simulink model "BEST2020_Autonomous_7thGraders"  (R2021a)
settings: Solver=ode23t  StartTime=0.0  StopTime=120.1  FixedStep=0.05  RelTol=1e-3  EnableMultiTasking=on
model workspace (MAT data in the model file):
  mapForSim : object (value not decoded)
  occGrid : robotics.BinaryOccupancyGrid (value not decoded)
values from neighbouring files (symbols this model uses):
  cellLevel = [0 0 0 1 0 0 0 0 0 0 0 0 0 0 0 0 0 0 1 0 0 ]    [BEST2020GameConfigAuto1.m]    (also in BEST2020GameConfigAuto2.m; BEST2020GameConfigAuto3.m)
  cellPose = [0.920 1.265;     1.035 1.380;     0.805 1.380;     0.920 0.920;     1.035 0.920;     0.805 0.920;     1.035 0.460;     0.920 0.575;     0.805 0.575;     0.575 0.000;     0.460 0.115;     0.345 0.000;     0.805 -0.460;     1.035 -0.460;     0.920 -0.460;     0.920 -0.805;     0.805 -0.920;     1.035 -1.035;     1.265 -1.265;     1.380 -1.380;     1.495 -1.265]    [BEST2020GameConfigAuto1.m]    (also in BEST2020GameConfigAuto2.m; BEST2020GameConfigAuto3.m)
  cellTypeArray = [0 0 0 0 0 0 0 0 0 0 0 0 0 0 0 0 0 0 0 0 0 ]    [BEST2020GameConfigAuto1.m]    (also in BEST2020GameConfigAuto2.m = [1 1 1 1 2 1 2 2 2 2 1 2 1 2 2 1 1 1 1 2 2 ]; BEST2020GameConfigAuto3.m = [0 0 1 1 0 0 0 1 2 0 0 1 0 0 1 0 0 2 2 0 1 ])
  isoPoses = [0.91 0;-0.91/2 0.91;-0.91/2 -0.91]    [BEST2020GameConfigAuto1.m]    (also in BEST2020GameConfigAuto2.m; BEST2020GameConfigAuto3.m)
  platformPoses = [0.91 0.91;1.37 -1.37]    [BEST2020GameConfigAuto1.m]    (also in BEST2020GameConfigAuto2.m; BEST2020GameConfigAuto3.m)
undefined symbols (not defined in the file or in its folder): FloorSurface, PlowSurface, Ref, RobotSurface, WallSurface, X, Y, Z
libraries: sm_lib x286, nesl_utility x157, simulink x72
(part 15 of 15)

== matlab function BEST2020_Autonomous_7thGraders/BEST Robotics 2020 Game (Double-Click)1/Cells/Object18/MATLAB Function ==
  settings: updateMethod=DISCRETE
  data: latch input; scoreLevel input; inuse input; target input; time input; objPoseX output; robotPoseX input; robotPoseY input; objPoseY output; latched output; initPose parameter; objId parameter; cellType output; endType output; cellTypeArray parameter; gameTime parameter; platformPoses parameter; cellLevel parameter
function [objPoseX, objPoseY, latched, cellType,endType] = latchObject(latch,scoreLevel, inuse, target, time, robotPoseX, robotPoseY, initPose, objId, cellTypeArray, gameTime, platformPoses, cellLevel)
persistent stateX stateY level pickup
if isempty(stateX)
    stateX=initPose(1);
    stateY=initPose(2);
    level=cellLevel;
    pickup=0;
end

if ~latch
     pickup=0;
    if level && ((stateX > platformPoses(1,1)-0.21 && stateX < platformPoses(1,1)+0.21...
            && stateY > platformPoses(1,2)-0.21 && stateY < platformPoses(1,2) +0.21) || ...
            (stateX > platformPoses(2,1)-0.21 && stateX < platformPoses(2,1)+0.21...
            && stateY > platformPoses(2,2)-0.21 && stateY < platformPoses(2,2) +0.21))
        latched=0.4;
    else
        level=0;
        latched=0;
    end
elseif pickup
    stateX=robotPoseX;
    stateY=robotPoseY;
    level=scoreLevel;
    latched=0.15 +level*0.4;
elseif ~inuse && latch && target == objId && ...
        sqrt((stateX-robotPoseX)^2+(stateY-robotPoseY)^2) < 0.08 && scoreLevel==level
    
        pickup=1;
        latched=0.15;
else
   if level && ((stateX > platformPoses(1,1)-0.21 && stateX < platformPoses(1,1)+0.21...
            && stateY > platformPoses(1,2)-0.21 && stateY < platformPoses(1,2) +0.21) || ...
            (stateX > platformPoses(2,1)-0.21 && stateX < platformPoses(2,1)+0.21...
            && stateY > platformPoses(2,2)-0.21 && stateY < platformPoses(2,2) +0.21))
        latched=0.4;
    else
        level=0;
        latched=0;
    end
end
if sqrt((stateX-robotPoseX)^2+(stateY-robotPoseY)^2) < 0.1 && scoreLevel==level
    cellType=cellTypeArray(objId);
else
    cellType=nan;
end

if time > gameTime
    endType=cellTypeArray(objId)+1;
else
    endType=0;
end

objPoseX=stateX;
objPoseY=stateY;

== matlab function BEST2020_Autonomous_7thGraders/BEST Robotics 2020 Game (Double-Click)1/Cells/Object19/MATLAB Function ==
  settings: updateMethod=DISCRETE
  data: latch input; scoreLevel input; inuse input; target input; time input; objPoseX output; robotPoseX input; robotPoseY input; objPoseY output; latched output; initPose parameter; objId parameter; cellType output; endType output; cellTypeArray parameter; gameTime parameter; platformPoses parameter; cellLevel parameter
function [objPoseX, objPoseY, latched, cellType,endType] = latchObject(latch,scoreLevel, inuse, target, time, robotPoseX, robotPoseY, initPose, objId, cellTypeArray, gameTime, platformPoses, cellLevel)
persistent stateX stateY level pickup
if isempty(stateX)
    stateX=initPose(1);
    stateY=initPose(2);
    level=cellLevel;
    pickup=0;
end

if ~latch
     pickup=0;
    if level && ((stateX > platformPoses(1,1)-0.21 && stateX < platformPoses(1,1)+0.21...
            && stateY > platformPoses(1,2)-0.21 && stateY < platformPoses(1,2) +0.21) || ...
            (stateX > platformPoses(2,1)-0.21 && stateX < platformPoses(2,1)+0.21...
            && stateY > platformPoses(2,2)-0.21 && stateY < platformPoses(2,2) +0.21))
        latched=0.4;
    else
        level=0;
        latched=0;
    end
elseif pickup
    stateX=robotPoseX;
    stateY=robotPoseY;
    level=scoreLevel;
    latched=0.15 +level*0.4;
elseif ~inuse && latch && target == objId && ...
        sqrt((stateX-robotPoseX)^2+(stateY-robotPoseY)^2) < 0.08 && scoreLevel==level
    
        pickup=1;
        latched=0.15;
else
   if level && ((stateX > platformPoses(1,1)-0.21 && stateX < platformPoses(1,1)+0.21...
            && stateY > platformPoses(1,2)-0.21 && stateY < platformPoses(1,2) +0.21) || ...
            (stateX > platformPoses(2,1)-0.21 && stateX < platformPoses(2,1)+0.21...
            && stateY > platformPoses(2,2)-0.21 && stateY < platformPoses(2,2) +0.21))
        latched=0.4;
    else
        level=0;
        latched=0;
    end
end
if sqrt((stateX-robotPoseX)^2+(stateY-robotPoseY)^2) < 0.1 && scoreLevel==level
    cellType=cellTypeArray(objId);
else
    cellType=nan;
end

if time > gameTime
    endType=cellTypeArray(objId)+1;
else
    endType=0;
end

objPoseX=stateX;
objPoseY=stateY;

== matlab function BEST2020_Autonomous_7thGraders/BEST Robotics 2020 Game (Double-Click)1/Cells/Object2/MATLAB Function ==
  settings: updateMethod=DISCRETE
  data: latch input; scoreLevel input; inuse input; target input; time input; objPoseX output; robotPoseX input; robotPoseY input; objPoseY output; latched output; initPose parameter; objId parameter; cellType output; endType output; cellTypeArray parameter; gameTime parameter; platformPoses parameter; cellLevel parameter
function [objPoseX, objPoseY, latched, cellType,endType] = latchObject(latch,scoreLevel, inuse, target, time, robotPoseX, robotPoseY, initPose, objId, cellTypeArray, gameTime, platformPoses, cellLevel)
persistent stateX stateY level pickup
if isempty(stateX)
    stateX=initPose(1);
    stateY=initPose(2);
    level=cellLevel;
    pickup=0;
end

if ~latch
     pickup=0;
    if level && ((stateX > platformPoses(1,1)-0.21 && stateX < platformPoses(1,1)+0.21...
            && stateY > platformPoses(1,2)-0.21 && stateY < platformPoses(1,2) +0.21) || ...
            (stateX > platformPoses(2,1)-0.21 && stateX < platformPoses(2,1)+0.21...
            && stateY > platformPoses(2,2)-0.21 && stateY < platformPoses(2,2) +0.21))
        latched=0.4;
    else
        level=0;
        latched=0;
    end
elseif pickup
    stateX=robotPoseX;
    stateY=robotPoseY;
    level=scoreLevel;
    latched=0.15 +level*0.4;
elseif ~inuse && latch && target == objId && ...
        sqrt((stateX-robotPoseX)^2+(stateY-robotPoseY)^2) < 0.08 && scoreLevel==level
    
        pickup=1;
        latched=0.15;
else
   if level && ((stateX > platformPoses(1,1)-0.21 && stateX < platformPoses(1,1)+0.21...
            && stateY > platformPoses(1,2)-0.21 && stateY < platformPoses(1,2) +0.21) || ...
            (stateX > platformPoses(2,1)-0.21 && stateX < platformPoses(2,1)+0.21...
            && stateY > platformPoses(2,2)-0.21 && stateY < platformPoses(2,2) +0.21))
        latched=0.4;
    else
        level=0;
        latched=0;
    end
end
if sqrt((stateX-robotPoseX)^2+(stateY-robotPoseY)^2) < 0.1 && scoreLevel==level
    cellType=cellTypeArray(objId);
else
    cellType=nan;
end

if time > gameTime
    endType=cellTypeArray(objId)+1;
else
    endType=0;
end

objPoseX=stateX;
objPoseY=stateY;

== matlab function BEST2020_Autonomous_7thGraders/BEST Robotics 2020 Game (Double-Click)1/Cells/Object20/MATLAB Function ==
  settings: updateMethod=DISCRETE
  data: latch input; scoreLevel input; inuse input; target input; time input; objPoseX output; robotPoseX input; robotPoseY input; objPoseY output; latched output; initPose parameter; objId parameter; cellType output; endType output; cellTypeArray parameter; gameTime parameter; platformPoses parameter; cellLevel parameter
function [objPoseX, objPoseY, latched, cellType,endType] = latchObject(latch,scoreLevel, inuse, target, time, robotPoseX, robotPoseY, initPose, objId, cellTypeArray, gameTime, platformPoses, cellLevel)
persistent stateX stateY level pickup
if isempty(stateX)
    stateX=initPose(1);
    stateY=initPose(2);
    level=cellLevel;
    pickup=0;
end

if ~latch
     pickup=0;
    if level && ((stateX > platformPoses(1,1)-0.21 && stateX < platformPoses(1,1)+0.21...
            && stateY > platformPoses(1,2)-0.21 && stateY < platformPoses(1,2) +0.21) || ...
            (stateX > platformPoses(2,1)-0.21 && stateX < platformPoses(2,1)+0.21...
            && stateY > platformPoses(2,2)-0.21 && stateY < platformPoses(2,2) +0.21))
        latched=0.4;
    else
        level=0;
        latched=0;
    end
elseif pickup
    stateX=robotPoseX;
    stateY=robotPoseY;
    level=scoreLevel;
    latched=0.15 +level*0.4;
elseif ~inuse && latch && target == objId && ...
        sqrt((stateX-robotPoseX)^2+(stateY-robotPoseY)^2) < 0.08 && scoreLevel==level
    
        pickup=1;
        latched=0.15;
else
   if level && ((stateX > platformPoses(1,1)-0.21 && stateX < platformPoses(1,1)+0.21...
            && stateY > platformPoses(1,2)-0.21 && stateY < platformPoses(1,2) +0.21) || ...
            (stateX > platformPoses(2,1)-0.21 && stateX < platformPoses(2,1)+0.21...
            && stateY > platformPoses(2,2)-0.21 && stateY < platformPoses(2,2) +0.21))
        latched=0.4;
    else
        level=0;
        latched=0;
    end
end
if sqrt((stateX-robotPoseX)^2+(stateY-robotPoseY)^2) < 0.1 && scoreLevel==level
    cellType=cellTypeArray(objId);
else
    cellType=nan;
end

if time > gameTime
    endType=cellTypeArray(objId)+1;
else
    endType=0;
end

objPoseX=stateX;
objPoseY=stateY;

== matlab function BEST2020_Autonomous_7thGraders/BEST Robotics 2020 Game (Double-Click)1/Cells/Object21/MATLAB Function ==
  settings: updateMethod=DISCRETE
  data: latch input; scoreLevel input; inuse input; target input; time input; objPoseX output; robotPoseX input; robotPoseY input; objPoseY output; latched output; initPose parameter; objId parameter; cellType output; endType output; cellTypeArray parameter; gameTime parameter; platformPoses parameter; cellLevel parameter
function [objPoseX, objPoseY, latched, cellType,endType] = latchObject(latch,scoreLevel, inuse, target, time, robotPoseX, robotPoseY, initPose, objId, cellTypeArray, gameTime, platformPoses, cellLevel)
persistent stateX stateY level pickup
if isempty(stateX)
    stateX=initPose(1);
    stateY=initPose(2);
    level=cellLevel;
    pickup=0;
end

if ~latch
     pickup=0;
    if level && ((stateX > platformPoses(1,1)-0.21 && stateX < platformPoses(1,1)+0.21...
            && stateY > platformPoses(1,2)-0.21 && stateY < platformPoses(1,2) +0.21) || ...
            (stateX > platformPoses(2,1)-0.21 && stateX < platformPoses(2,1)+0.21...
            && stateY > platformPoses(2,2)-0.21 && stateY < platformPoses(2,2) +0.21))
        latched=0.4;
    else
        level=0;
        latched=0;
    end
elseif pickup
    stateX=robotPoseX;
    stateY=robotPoseY;
    level=scoreLevel;
    latched=0.15 +level*0.4;
elseif ~inuse && latch && target == objId && ...
        sqrt((stateX-robotPoseX)^2+(stateY-robotPoseY)^2) < 0.08 && scoreLevel==level
    
        pickup=1;
        latched=0.15;
else
   if level && ((stateX > platformPoses(1,1)-0.21 && stateX < platformPoses(1,1)+0.21...
            && stateY > platformPoses(1,2)-0.21 && stateY < platformPoses(1,2) +0.21) || ...
            (stateX > platformPoses(2,1)-0.21 && stateX < platformPoses(2,1)+0.21...
            && stateY > platformPoses(2,2)-0.21 && stateY < platformPoses(2,2) +0.21))
        latched=0.4;
    else
        level=0;
        latched=0;
    end
end
if sqrt((stateX-robotPoseX)^2+(stateY-robotPoseY)^2) < 0.1 && scoreLevel==level
    cellType=cellTypeArray(objId);
else
    cellType=nan;
end

if time > gameTime
    endType=cellTypeArray(objId)+1;
else
    endType=0;
end

objPoseX=stateX;
objPoseY=stateY;

== matlab function BEST2020_Autonomous_7thGraders/BEST Robotics 2020 Game (Double-Click)1/Cells/Object3/MATLAB Function ==
  settings: updateMethod=DISCRETE
  data: latch input; scoreLevel input; inuse input; target input; time input; objPoseX output; robotPoseX input; robotPoseY input; objPoseY output; latched output; initPose parameter; objId parameter; cellType output; endType output; cellTypeArray parameter; gameTime parameter; platformPoses parameter; cellLevel parameter
function [objPoseX, objPoseY, latched, cellType,endType] = latchObject(latch,scoreLevel, inuse, target, time, robotPoseX, robotPoseY, initPose, objId, cellTypeArray, gameTime, platformPoses, cellLevel)
persistent stateX stateY level pickup
if isempty(stateX)
    stateX=initPose(1);
    stateY=initPose(2);
    level=cellLevel;
    pickup=0;
end

if ~latch
     pickup=0;
    if level && ((stateX > platformPoses(1,1)-0.21 && stateX < platformPoses(1,1)+0.21...
            && stateY > platformPoses(1,2)-0.21 && stateY < platformPoses(1,2) +0.21) || ...
            (stateX > platformPoses(2,1)-0.21 && stateX < platformPoses(2,1)+0.21...
            && stateY > platformPoses(2,2)-0.21 && stateY < platformPoses(2,2) +0.21))
        latched=0.4;
    else
        level=0;
        latched=0;
    end
elseif pickup
    stateX=robotPoseX;
    stateY=robotPoseY;
    level=scoreLevel;
    latched=0.15 +level*0.4;
elseif ~inuse && latch && target == objId && ...
        sqrt((stateX-robotPoseX)^2+(stateY-robotPoseY)^2) < 0.08 && scoreLevel==level
    
        pickup=1;
        latched=0.15;
else
   if level && ((stateX > platformPoses(1,1)-0.21 && stateX < platformPoses(1,1)+0.21...
            && stateY > platformPoses(1,2)-0.21 && stateY < platformPoses(1,2) +0.21) || ...
            (stateX > platformPoses(2,1)-0.21 && stateX < platformPoses(2,1)+0.21...
            && stateY > platformPoses(2,2)-0.21 && stateY < platformPoses(2,2) +0.21))
        latched=0.4;
    else
        level=0;
        latched=0;
    end
end
if sqrt((stateX-robotPoseX)^2+(stateY-robotPoseY)^2) < 0.1 && scoreLevel==level
    cellType=cellTypeArray(objId);
else
    cellType=nan;
end

if time > gameTime
    endType=cellTypeArray(objId)+1;
else
    endType=0;
end

objPoseX=stateX;
objPoseY=stateY;

== matlab function BEST2020_Autonomous_7thGraders/BEST Robotics 2020 Game (Double-Click)1/Cells/Object4/MATLAB Function ==
  settings: updateMethod=DISCRETE
  data: latch input; scoreLevel input; inuse input; target input; time input; objPoseX output; robotPoseX input; robotPoseY input; objPoseY output; latched output; initPose parameter; objId parameter; cellType output; endType output; cellTypeArray parameter; gameTime parameter; platformPoses parameter; cellLevel parameter
function [objPoseX, objPoseY, latched, cellType,endType] = latchObject(latch,scoreLevel, inuse, target, time, robotPoseX, robotPoseY, initPose, objId, cellTypeArray, gameTime, platformPoses, cellLevel)
persistent stateX stateY level pickup
if isempty(stateX)
    stateX=initPose(1);
    stateY=initPose(2);
    level=cellLevel;
    pickup=0;
end

if ~latch
     pickup=0;
    if level && ((stateX > platformPoses(1,1)-0.21 && stateX < platformPoses(1,1)+0.21...
            && stateY > platformPoses(1,2)-0.21 && stateY < platformPoses(1,2) +0.21) || ...
            (stateX > platformPoses(2,1)-0.21 && stateX < platformPoses(2,1)+0.21...
            && stateY > platformPoses(2,2)-0.21 && stateY < platformPoses(2,2) +0.21))
        latched=0.4;
    else
        level=0;
        latched=0;
    end
elseif pickup
    stateX=robotPoseX;
    stateY=robotPoseY;
    level=scoreLevel;
    latched=0.15 +level*0.4;
elseif ~inuse && latch && target == objId && ...
        sqrt((stateX-robotPoseX)^2+(stateY-robotPoseY)^2) < 0.08 && scoreLevel==level
    
        pickup=1;
        latched=0.15;
else
   if level && ((stateX > platformPoses(1,1)-0.21 && stateX < platformPoses(1,1)+0.21...
            && stateY > platformPoses(1,2)-0.21 && stateY < platformPoses(1,2) +0.21) || ...
            (stateX > platformPoses(2,1)-0.21 && stateX < platformPoses(2,1)+0.21...
            && stateY > platformPoses(2,2)-0.21 && stateY < platformPoses(2,2) +0.21))
        latched=0.4;
    else
        level=0;
        latched=0;
    end
end
if sqrt((stateX-robotPoseX)^2+(stateY-robotPoseY)^2) < 0.1 && scoreLevel==level
    cellType=cellTypeArray(objId);
else
    cellType=nan;
end

if time > gameTime
    endType=cellTypeArray(objId)+1;
else
    endType=0;
end

objPoseX=stateX;
objPoseY=stateY;

== matlab function BEST2020_Autonomous_7thGraders/BEST Robotics 2020 Game (Double-Click)1/Cells/Object5/MATLAB Function ==
  settings: updateMethod=DISCRETE
  data: latch input; scoreLevel input; inuse input; target input; time input; objPoseX output; robotPoseX input; robotPoseY input; objPoseY output; latched output; initPose parameter; objId parameter; cellType output; endType output; cellTypeArray parameter; gameTime parameter; platformPoses parameter; cellLevel parameter
function [objPoseX, objPoseY, latched, cellType,endType] = latchObject(latch,scoreLevel, inuse, target, time, robotPoseX, robotPoseY, initPose, objId, cellTypeArray, gameTime, platformPoses, cellLevel)
persistent stateX stateY level pickup
if isempty(stateX)
    stateX=initPose(1);
    stateY=initPose(2);
    level=cellLevel;
    pickup=0;
end

if ~latch
     pickup=0;
    if level && ((stateX > platformPoses(1,1)-0.21 && stateX < platformPoses(1,1)+0.21...
            && stateY > platformPoses(1,2)-0.21 && stateY < platformPoses(1,2) +0.21) || ...
            (stateX > platformPoses(2,1)-0.21 && stateX < platformPoses(2,1)+0.21...
            && stateY > platformPoses(2,2)-0.21 && stateY < platformPoses(2,2) +0.21))
        latched=0.4;
    else
        level=0;
        latched=0;
    end
elseif pickup
    stateX=robotPoseX;
    stateY=robotPoseY;
    level=scoreLevel;
    latched=0.15 +level*0.4;
elseif ~inuse && latch && target == objId && ...
        sqrt((stateX-robotPoseX)^2+(stateY-robotPoseY)^2) < 0.08 && scoreLevel==level
    
        pickup=1;
        latched=0.15;
else
   if level && ((stateX > platformPoses(1,1)-0.21 && stateX < platformPoses(1,1)+0.21...
            && stateY > platformPoses(1,2)-0.21 && stateY < platformPoses(1,2) +0.21) || ...
            (stateX > platformPoses(2,1)-0.21 && stateX < platformPoses(2,1)+0.21...
            && stateY > platformPoses(2,2)-0.21 && stateY < platformPoses(2,2) +0.21))
        latched=0.4;
    else
        level=0;
        latched=0;
    end
end
if sqrt((stateX-robotPoseX)^2+(stateY-robotPoseY)^2) < 0.1 && scoreLevel==level
    cellType=cellTypeArray(objId);
else
    cellType=nan;
end

if time > gameTime
    endType=cellTypeArray(objId)+1;
else
    endType=0;
end

objPoseX=stateX;
objPoseY=stateY;

== matlab function BEST2020_Autonomous_7thGraders/BEST Robotics 2020 Game (Double-Click)1/Cells/Object6/MATLAB Function ==
  settings: updateMethod=DISCRETE
  data: latch input; scoreLevel input; inuse input; target input; time input; objPoseX output; robotPoseX input; robotPoseY input; objPoseY output; latched output; initPose parameter; objId parameter; cellType output; endType output; cellTypeArray parameter; gameTime parameter; platformPoses parameter; cellLevel parameter
function [objPoseX, objPoseY, latched, cellType,endType] = latchObject(latch,scoreLevel, inuse, target, time, robotPoseX, robotPoseY, initPose, objId, cellTypeArray, gameTime, platformPoses, cellLevel)
persistent stateX stateY level pickup
if isempty(stateX)
    stateX=initPose(1);
    stateY=initPose(2);
    level=cellLevel;
    pickup=0;
end

if ~latch
     pickup=0;
    if level && ((stateX > platformPoses(1,1)-0.21 && stateX < platformPoses(1,1)+0.21...
            && stateY > platformPoses(1,2)-0.21 && stateY < platformPoses(1,2) +0.21) || ...
            (stateX > platformPoses(2,1)-0.21 && stateX < platformPoses(2,1)+0.21...
            && stateY > platformPoses(2,2)-0.21 && stateY < platformPoses(2,2) +0.21))
        latched=0.4;
    else
        level=0;
        latched=0;
    end
elseif pickup
    stateX=robotPoseX;
    stateY=robotPoseY;
    level=scoreLevel;
    latched=0.15 +level*0.4;
elseif ~inuse && latch && target == objId && ...
        sqrt((stateX-robotPoseX)^2+(stateY-robotPoseY)^2) < 0.08 && scoreLevel==level
    
        pickup=1;
        latched=0.15;
else
   if level && ((stateX > platformPoses(1,1)-0.21 && stateX < platformPoses(1,1)+0.21...
            && stateY > platformPoses(1,2)-0.21 && stateY < platformPoses(1,2) +0.21) || ...
            (stateX > platformPoses(2,1)-0.21 && stateX < platformPoses(2,1)+0.21...
            && stateY > platformPoses(2,2)-0.21 && stateY < platformPoses(2,2) +0.21))
        latched=0.4;
    else
        level=0;
        latched=0;
    end
end
if sqrt((stateX-robotPoseX)^2+(stateY-robotPoseY)^2) < 0.1 && scoreLevel==level
    cellType=cellTypeArray(objId);
else
    cellType=nan;
end

if time > gameTime
    endType=cellTypeArray(objId)+1;
else
    endType=0;
end

objPoseX=stateX;
objPoseY=stateY;

== matlab function BEST2020_Autonomous_7thGraders/BEST Robotics 2020 Game (Double-Click)1/Cells/Object7/MATLAB Function ==
  settings: updateMethod=DISCRETE
  data: latch input; scoreLevel input; inuse input; target input; time input; objPoseX output; robotPoseX input; robotPoseY input; objPoseY output; latched output; initPose parameter; objId parameter; cellType output; endType output; cellTypeArray parameter; gameTime parameter; platformPoses parameter; cellLevel parameter
function [objPoseX, objPoseY, latched, cellType,endType] = latchObject(latch,scoreLevel, inuse, target, time, robotPoseX, robotPoseY, initPose, objId, cellTypeArray, gameTime, platformPoses, cellLevel)
persistent stateX stateY level pickup
if isempty(stateX)
    stateX=initPose(1);
    stateY=initPose(2);
    level=cellLevel;
    pickup=0;
end

if ~latch
     pickup=0;
    if level && ((stateX > platformPoses(1,1)-0.21 && stateX < platformPoses(1,1)+0.21...
            && stateY > platformPoses(1,2)-0.21 && stateY < platformPoses(1,2) +0.21) || ...
            (stateX > platformPoses(2,1)-0.21 && stateX < platformPoses(2,1)+0.21...
            && stateY > platformPoses(2,2)-0.21 && stateY < platformPoses(2,2) +0.21))
        latched=0.4;
    else
        level=0;
        latched=0;
    end
elseif pickup
    stateX=robotPoseX;
    stateY=robotPoseY;
    level=scoreLevel;
    latched=0.15 +level*0.4;
elseif ~inuse && latch && target == objId && ...
        sqrt((stateX-robotPoseX)^2+(stateY-robotPoseY)^2) < 0.08 && scoreLevel==level
    
        pickup=1;
        latched=0.15;
else
   if level && ((stateX > platformPoses(1,1)-0.21 && stateX < platformPoses(1,1)+0.21...
            && stateY > platformPoses(1,2)-0.21 && stateY < platformPoses(1,2) +0.21) || ...
            (stateX > platformPoses(2,1)-0.21 && stateX < platformPoses(2,1)+0.21...
            && stateY > platformPoses(2,2)-0.21 && stateY < platformPoses(2,2) +0.21))
        latched=0.4;
    else
        level=0;
        latched=0;
    end
end
if sqrt((stateX-robotPoseX)^2+(stateY-robotPoseY)^2) < 0.1 && scoreLevel==level
    cellType=cellTypeArray(objId);
else
    cellType=nan;
end

if time > gameTime
    endType=cellTypeArray(objId)+1;
else
    endType=0;
end

objPoseX=stateX;
objPoseY=stateY;
